simulink model "VFlexP"  (R2024a)
settings: Solver=ode23tb  StartTime=0.0  StopTime=3  FixedStep=1e-5
model workspace (MAT data in the model file):
  DCop_DCBUCK : object (value not decoded)
  Grid_CCVSC_idx = [2; 3; 4; 5; 6; 7; 8; 9; 10; 11; 12]
  Grid_CCVSCs = 1
  Grid_CCVSCs_buses = 1
  Grid_CCVSCs_toM = [0 1 0 0 0 0 0 0 0 0 0 0 ... (781 elements, 71x11)]
  Grid_C_Lines = [0 0]
  Grid_Cbuses = [0.00666666666667 0.00666666666667 0.00666666666667]
  Grid_DC : object (value not decoded)
  Grid_DCop_DCBUCK : object (value not decoded)
  Grid_DCop_DC_PES : object (value not decoded)
  Grid_DFIGs = 1
  Grid_DFIGs_buses = 1
  Grid_DGs : string (value not decoded)
  Grid_From_buses = [1 2]
  Grid_GFls = 1
  Grid_GFls_buses = 1
  Grid_GFr_idx = 1
  Grid_GFrs = 1
  Grid_GFrs_buses = 1
  Grid_GFrs_toM = [1; 0; 0]
  Grid_IG_idx = 2
  Grid_IGs = 1
  Grid_IGs_buses = 1
  Grid_IGs_toM = [0; 1]
  Grid_L_Lines = [0.05 0.05]
  Grid_L_Loads = 0
  Grid_Lines_fromM : object (value not decoded)
  Grid_Lines_toM : object (value not decoded)
  Grid_Load_buses = []
  Grid_Load_busesDC = []
  Grid_MSGs = 1
  Grid_MSGs_buses = 1
  Grid_Nbuses = 3
  Grid_PQ_gen = 3
  Grid_Ploads = []
  Grid_PloadsDC = []
  Grid_Ps_lf = -0.138475313333
  Grid_Qloads = []
  Grid_Qs_lf = 0.00594619333333
  Grid_R_Lines = [0.005 0.005]
  Grid_R_Loads = 0
  Grid_R_Loads_DC = 0
  Grid_Rcf = [150 150 150]
  Grid_SCs = 1
  Grid_SCs_buses = 1
  Grid_SG_idx = 1
  Grid_SGs = 1
  Grid_SGs_buses = 1
  Grid_SGs_toM = [1; 0]
  Grid_To_buses = [2 3]
  Grid_VCVSC_idx = [1; 2; 3; 4; 5; 6; 7; 8; 9; 10; 11; 12]
  Grid_VCVSCs = 1
  Grid_VCVSCs_buses = [1; 2; 3; 6; 8; 9; 12; 58; 59; 60; 63; 65]
  Grid_VCVSCs_toM = [1 0 0 0 0 0 0 0 0 0 0 0 ... (852 elements, 71x12)]
  Grid_VSM_idx = 2
  Grid_VSMs = 1
  Grid_VSMs_buses = 1
  Grid_VSMs_toM = [0; 1]
  Grid_admitt_matrix = [1.9801990198-19.801979198i  -1.9801980198+19.801980198i; -1.9801980198+19.801980198i  1.9801990198-19.801979198i]
  Grid_admitt_matrix_noloads = [1.9801990198-19.801979198i  -1.9801980198+19.801980198i; -1.9801980198+19.801980198i  1.9801990198-19.801979198i]
  Grid_bus = [1; 2; 3]
  Grid_busDC_complexity = 1
  Grid_busDC_complexity_PF = 2
  Grid_bus_complexity = [1 1 1]
  Grid_bus_complexity_PF = [1 1 1]
  Grid_buses_lf = 1
  Grid_conductance_matrix = 0.00666666666667
  Grid_conductance_matrix_noloads = 0.00666666666667
  Grid_fref : object (value not decoded)
  Grid_gen_static_params : mBase (value not decoded)
  Grid_iPs_lf = -7.22150378958
  Grid_iQs_lf = 168.17482109
  Grid_iadmitt_matrix = [250000.001075-249999.987531i  249999.998575-250000.012531i; 249999.998575-250000.012531i  250000.001075-249999.987531i]
  Grid_iadmitt_matrix_noloads = [250000.001075-249999.987531i  249999.998575-250000.012531i; 249999.998575-250000.012531i  250000.001075-249999.987531i]
  Grid_iconductance_matrix = 150
  Grid_iconductance_matrix_noloads = 150
  Grid_init_OK_bool = 1
  Grid_intconv_PF : object (value not decoded)
  Grid_lf_op : op_report (value not decoded)
  Grid_lineDC_complexity = []
  Grid_lineDC_complexity_PF = []
  Grid_line_complexity = [1 1]
  Grid_line_complexity_PF = [3 3]
  Grid_loadDC_complexity = []
  Grid_loadDC_complexity_PF = []
  Grid_load_complexity = []
  Grid_load_complexity_PF = []
  Grid_opDC_CCVSC : object (value not decoded)
  Grid_opDC_VSM : object (value not decoded)
  Grid_opGFr : object (value not decoded)
  Grid_opVCVSC : object (value not decoded)
  Grid_op_CCVSC : object (value not decoded)
  Grid_op_IG : object (value not decoded)
  Grid_op_SG : object (value not decoded)
  Grid_op_VSM : object (value not decoded)
  Grid_shift_lines = [0 0]
  Grid_tap_lines = [1 1]
  Grid_v_buses_mod = [1 1.0001218564 1]
  LinsysParamChangeStruct : Param1 (value not decoded)
  Lline = 0.01
  Rline = 1e-05
  linsys : object (value not decoded)
symbols that are objects in the model workspace (value not decoded): Grid_DCop_DC_PES, Grid_DCop_DCBUCK, Grid_op_CCVSC, Grid_op_IG, Grid_op_SG, Grid_op_VSM, Grid_opDC_CCVSC, Grid_opDC_VSM, Grid_opGFr, Grid_opVCVSC
undefined symbols (not defined in the file or in its folder): block_buses_DC, block_idx, CCVSC_idx, Cf, costs, costs2, DFIGs_nodes, DiscIntNeverNeededParam, entity, Fb, Fi, From_nodes, Grid_op_DFIG, Grid_op_DFIG_PQ, Grid_op_MSG, Grid_op_SC, Grid_op_VCVSC, Kic, Kiv, Kpc, Kpv, last_send, Lc, Lf, m, Matrix_flux_to_i, mD, mp, MSGs_buses, Nbuses_DC, nq, op_VCVSC, Psche, Rc, Rf, rkq1, rkq2, SCs_buses, SCs_nodes, sec_control_structure, set_DG_up, set_extra_satur, set_sending_cost, SGs_buses, SGs_nodes, Tf, To_nodes, VI_L, VI_R, WOF_Tf, xkq1, xkq2
libraries: simulink x447, eeGeneralControl x5
(part 10 of 30)

== system VFlexP/Grid/Dynamic/Generators/SG/Electromagnetic ==
  note: 1) Add Subsystem or Model blocks as valid variant choices.
      | 2) You cannot connect blocks at this level. At simulation, connectivity is automatically
      | determined, based on the active variant and port name matching.
  vsd : Inport
  vsq : Inport  Port=2
  vfd : Inport  Port=3
  ws : Inport  Port=4
  order 2 : Subsystem  VariantControl=order 2
  order 8 : Subsystem  VariantControl=order 8
  order 8 nomatrix : Subsystem  VariantControl=order 1  mask{Lssd_pu=Lssd_pu, Lssq_pu=Lssq_pu, Lmd_pu=Lmd_pu, Lmq_pu=Lmq_pu, Lfd_pu=Lfd_pu, Lkd1_pu=Lkd1_pu, Lkd2_pu=Lkd2_pu, Lkq1_pu=Lkq1_pu, Lkq2_pu=Lkq2_pu, Lkq3_pu=Lkq3_pu}
      mask init:
      | for i=1:length(Lssd_pu)
      |         Lssd = Lssd_pu(i);
      |         Lssq = Lssq_pu(i);
      |         Lmd = Lmd_pu(i);
      |         Lmq = Lmq_pu(i);
      |         Lfd = Lfd_pu(i);
      |         Lkd1 = Lkd1_pu(i);
      |         Lkd2 = Lkd2_pu(i);
      |         Lkq1 = Lkq1_pu(i);
      |         Lkq2 = Lkq2_pu(i);
      |         Lkq3 = Lkq3_pu(i);
      |         Matrix_flux_to_i(:,:,i) = [(0 - (Lfd(i)*Lmd(i)^2 + Lkd2(i)*Lmd(i)^2 - Lmd(i)^3 - Lfd(i)*Lkd1(i)*Lkd2(i))/(2*Lmd(i)^4 - Lkd1(i)*Lmd(i)^3 - 2*Lkd2(i)*Lmd(i)^3 - Lmd(i)^3*Lssd(i) - 2*Lfd(i)*Lmd(i)^3 + Lfd(i)*Lkd1(i)*Lmd(i)^2 + Lfd(i)*Lkd2(i)*Lmd(i)^2 + Lkd1(i)*Lkd2(i)*Lmd(i)^2 + Lfd(i)*Lmd(i)^2*Lssd(i) + Lkd2(i)*Lmd(i)^2*Lssd(i) - Lfd(i)*Lkd1(i)*Lkd2(i)*Lssd(i))),  + 0,  + (0 + (Lkd1(i)*Lmd(i)^2 + Lkd2(i)*Lmd(i)^2 - Lmd(i)^3 - Lkd1(i)*Lkd2(i)*Lmd(i))/(2*Lmd(i)^4 - Lkd1(i)*Lmd(i)^3 - 2*Lkd2(i)*Lmd(i)^3 - Lmd(i)^3*Lssd(i) - 2*Lfd(i)*Lmd(i)^3 + Lfd(i)*Lkd1(i)*Lmd(i)^2 + Lfd(i)*Lkd2(i)*Lmd(i)^2 + Lkd1(i)*Lkd2(i)*Lmd(i)^2 + Lfd(i)*Lmd(i)^2*Lssd(i) + Lkd2(i)*Lmd(i)^2*Lssd(i) - Lfd(i)*Lkd1(i)*Lkd2(i)*Lssd(i))),  + (0 + (Lfd(i)*Lmd(i)^2 + Lkd2(i)*Lmd(i)^2 - Lmd(i)^3 - Lfd(i)*Lkd2(i)*Lmd(i))/(2*Lmd(i)^4 - Lkd1(i)*Lmd(i)^3 - 2*Lkd2(i)*Lmd(i)^3 - Lmd(i)^3*Lssd(i) - 2*Lfd(i)*Lmd(i)^3 + Lfd(i)*Lkd1(i)*Lmd(i)^2 + Lfd(i)*Lkd2(i)*Lmd(i)^2 + Lkd1(i)*Lkd2(i)*Lmd(i)^2 + Lfd(i)*Lmd(i)^2*Lssd(i) + Lkd2(i)*Lmd(i)^2*Lssd(i) - Lfd(i)*Lkd1(i)*Lkd2(i)*Lssd(i))),  + (0 + (Lfd(i)*Lmd(i)^2 - Lfd(i)*Lkd1(i)*Lmd(i))/(2*Lmd(i)^4 - Lkd1(i)*Lmd(i)^3 - 2*Lkd2(i)*Lmd(i)^3 - Lmd(i)^3*Lssd(i) - 2*Lfd(i)*Lmd(i)^3 + Lfd(i)*Lkd1(i)*Lmd(i)^2 + Lfd(i)*Lkd2(i)*Lmd(i)^2 + Lkd1(i)*Lkd2(i)*Lmd(i)^2 + Lfd(i)*Lmd(i)^2*Lssd(i) + Lkd2(i)*Lmd(i)^2*Lssd(i) - Lfd(i)*Lkd1(i)*Lkd2(i)*Lssd(i))),  + 0,  + 0,  + 0, ; 0,  + (0 - (Lkq1(i)*Lmq(i)^2 + Lkq2(i)*Lmq(i)^2 + Lkq3(i)*Lmq(i)^2 - 2*Lmq(i)^3 - Lkq1(i)*Lkq2(i)*Lkq3(i))/(3*Lmq(i)^4 - 2*Lkq2(i)*Lmq(i)^3 - 2*Lkq3(i)*Lmq(i)^3 - 2*Lmq(i)^3*Lssq(i) - 2*Lkq1(i)*Lmq(i)^3 + Lkq1(i)*Lkq2(i)*Lmq(i)^2 + Lkq1(i)*Lkq3(i)*Lmq(i)^2 + Lkq2(i)*Lkq3(i)*Lmq(i)^2 + Lkq1(i)*Lmq(i)^2*Lssq(i) + Lkq2(i)*Lmq(i)^2*Lssq(i) + Lkq3(i)*Lmq(i)^2*Lssq(i) - Lkq1(i)*Lkq2(i)*Lkq3(i)*Lssq(i))),  + 0,  + 0,  + 0,  + (0 - (3*Lmq(i)^3 - 2*Lkq2(i)*Lmq(i)^2 - 2*Lkq3(i)*Lmq(i)^2 - 2*Lkq1(i)*Lmq(i)^2 + Lkq1(i)*Lkq2(i)*Lmq(i) + Lkq1(i)*Lkq3(i)*Lmq(i) + Lkq2(i)*Lkq3(i)*Lmq(i))/(3*Lmq(i)^4 - 2*Lkq2(i)*Lmq(i)^3 - 2*Lkq3(i)*Lmq(i)^3 - 2*Lmq(i)^3*Lssq(i) - 2*Lkq1(i)*Lmq(i)^3 + Lkq1(i)*Lkq2(i)*Lmq(i)^2 + Lkq1(i)*Lkq3(i)*Lmq(i)^2 + Lkq2(i)*Lkq3(i)*Lmq(i)^2 + Lkq1(i)*Lmq(i)^2*Lssq(i) + Lkq2(i)*Lmq(i)^2*Lssq(i) + Lkq3(i)*Lmq(i)^2*Lssq(i) - Lkq1(i)*Lkq2(i)*Lkq3(i)*Lssq(i))),  + 0,  + 0, ; (0 - (Lkd2(i)*Lmd(i)^2 - Lkd1(i)*Lkd2(i)*Lmd(i))/(2*Lmd(i)^4 - Lkd1(i)*Lmd(i)^3 - 2*Lkd2(i)*Lmd(i)^3 - Lmd(i)^3*Lssd(i) - 2*Lfd(i)*Lmd(i)^3 + Lfd(i)*Lkd1(i)*Lmd(i)^2 + Lfd(i)*Lkd2(i)*Lmd(i)^2 + Lkd1(i)*Lkd2(i)*Lmd(i)^2 + Lfd(i)*Lmd(i)^2*Lssd(i) + Lkd2(i)*Lmd(i)^2*Lssd(i) - Lfd(i)*Lkd1(i)*Lkd2(i)*Lssd(i))),  + 0,  + (0 + (Lkd1(i)*Lmd(i)^2 + Lkd2(i)*Lmd(i)^2 + Lmd(i)^2*Lssd(i) - 2*Lmd(i)^3 - Lkd1(i)*Lkd2(i)*Lssd(i))/(2*Lmd(i)^4 - Lkd1(i)*Lmd(i)^3 - 2*Lkd2(i)*Lmd(i)^3 - Lmd(i)^3*Lssd(i) - 2*Lfd(i)*Lmd(i)^3 + Lfd(i)*Lkd1(i)*Lmd(i)^2 + Lfd(i)*Lkd2(i)*Lmd(i)^2 + Lkd1(i)*Lkd2(i)*Lmd(i)^2 + Lfd(i)*Lmd(i)^2*Lssd(i) + Lkd2(i)*Lmd(i)^2*Lssd(i) - Lfd(i)*Lkd1(i)*Lkd2(i)*Lssd(i))),  + (0 - (Lkd2(i)*Lmd(i)^2 - Lkd2(i)*Lssd(i)*Lmd(i))/(2*Lmd(i)^4 - Lkd1(i)*Lmd(i)^3 - 2*Lkd2(i)*Lmd(i)^3 - Lmd(i)^3*Lssd(i) - 2*Lfd(i)*Lmd(i)^3 + Lfd(i)*Lkd1(i)*Lmd(i)^2 + Lfd(i)*Lkd2(i)*Lmd(i)^2 + Lkd1(i)*Lkd2(i)*Lmd(i)^2 + Lfd(i)*Lmd(i)^2*Lssd(i) + Lkd2(i)*Lmd(i)^2*Lssd(i) - Lfd(i)*Lkd1(i)*Lkd2(i)*Lssd(i))),  + (0 - (Lkd1(i)*Lmd(i)^2 + Lmd(i)^2*Lssd(i) - 2*Lmd(i)^3)/(2*Lmd(i)^4 - Lkd1(i)*Lmd(i)^3 - 2*Lkd2(i)*Lmd(i)^3 - Lmd(i)^3*Lssd(i) - 2*Lfd(i)*Lmd(i)^3 + Lfd(i)*Lkd1(i)*Lmd(i)^2 + Lfd(i)*Lkd2(i)*Lmd(i)^2 + Lkd1(i)*Lkd2(i)*Lmd(i)^2 + Lfd(i)*Lmd(i)^2*Lssd(i) + Lkd2(i)*Lmd(i)^2*Lssd(i) - Lfd(i)*Lkd1(i)*Lkd2(i)*Lssd(i))),  + 0,  + 0,  + 0, ; (0 - (Lfd(i)*Lmd(i)^2 + Lkd2(i)*Lmd(i)^2 - Lmd(i)^3 - Lfd(i)*Lkd2(i)*Lmd(i))/(2*Lmd(i)^4 - Lkd1(i)*Lmd(i)^3 - 2*Lkd2(i)*Lmd(i)^3 - Lmd(i)^3*Lssd(i) - 2*Lfd(i)*Lmd(i)^3 + Lfd(i)*Lkd1(i)*Lmd(i)^2 + Lfd(i)*Lkd2(i)*Lmd(i)^2 + Lkd1(i)*Lkd2(i)*Lmd(i)^2 + Lfd(i)*Lmd(i)^2*Lssd(i) + Lkd2(i)*Lmd(i)^2*Lssd(i) - Lfd(i)*Lkd1(i)*Lkd2(i)*Lssd(i))),  + 0,  + (0 - (Lkd2(i)*Lmd(i)^2 + Lmd(i)^2*Lssd(i) - Lmd(i)^3 - Lkd2(i)*Lmd(i)*Lssd(i))/(2*Lmd(i)^4 - Lkd1(i)*Lmd(i)^3 - 2*Lkd2(i)*Lmd(i)^3 - Lmd(i)^3*Lssd(i) - 2*Lfd(i)*Lmd(i)^3 + Lfd(i)*Lkd1(i)*Lmd(i)^2 + Lfd(i)*Lkd2(i)*Lmd(i)^2 + Lkd1(i)*Lkd2(i)*Lmd(i)^2 + Lfd(i)*Lmd(i)^2*Lssd(i) + Lkd2(i)*Lmd(i)^2*Lssd(i) - Lfd(i)*Lkd1(i)*Lkd2(i)*Lssd(i))),  + (0 + (Lfd(i)*Lmd(i)^2 + Lkd2(i)*Lmd(i)^2 - Lmd(i)^3 - Lfd(i)*Lkd2(i)*Lssd(i))/(2*Lmd(i)^4 - Lkd1(i)*Lmd(i)^3 - 2*Lkd2(i)*Lmd(i)^3 - Lmd(i)^3*Lssd(i) - 2*Lfd(i)*Lmd(i)^3 + Lfd(i)*Lkd1(i)*Lmd(i)^2 + Lfd(i)*Lkd2(i)*Lmd(i)^2 + Lkd1(i)*Lkd2(i)*Lmd(i)^2 + Lfd(i)*Lmd(i)^2*Lssd(i) + Lkd2(i)*Lmd(i)^2*Lssd(i) - Lfd(i)*Lkd1(i)*Lkd2(i)*Lssd(i))),  + (0 - (Lfd(i)*Lmd(i)^2 - Lfd(i)*Lssd(i)*Lmd(i))/(2*Lmd(i)^4 - Lkd1(i)*Lmd(i)^3 - 2*Lkd2(i)*Lmd(i)^3 - Lmd(i)^3*Lssd(i) - 2*Lfd(i)*Lmd(i)^3 + Lfd(i)*Lkd1(i)*Lmd(i)^2 + Lfd(i)*Lkd2(i)*Lmd(i)^2 + Lkd1(i)*Lkd2(i)*Lmd(i)^2 + Lfd(i)*Lmd(i)^2*Lssd(i) + Lkd2(i)*Lmd(i)^2*Lssd(i) - Lfd(i)*Lkd1(i)*Lkd2(i)*Lssd(i))),  + 0,  + 0,  + 0, ; (0 - (Lfd(i)*Lmd(i)^2 + Lkd1(i)*Lmd(i)^2 - Lmd(i)^3 - Lfd(i)*Lkd1(i)*Lmd(i))/(2*Lmd(i)^4 - Lkd1(i)*Lmd(i)^3 - 2*Lkd2(i)*Lmd(i)^3 - Lmd(i)^3*Lssd(i) - 2*Lfd(i)*Lmd(i)^3 + Lfd(i)*Lkd1(i)*Lmd(i)^2 + Lfd(i)*Lkd2(i)*Lmd(i)^2 + Lkd1(i)*Lkd2(i)*Lmd(i)^2 + Lfd(i)*Lmd(i)^2*Lssd(i) + Lkd2(i)*Lmd(i)^2*Lssd(i) - Lfd(i)*Lkd1(i)*Lkd2(i)*Lssd(i))),  + 0,  + (0 - (Lkd1(i)*Lmd(i)^2 + Lmd(i)^2*Lssd(i) - Lmd(i)^3 - Lkd1(i)*Lmd(i)*Lssd(i))/(2*Lmd(i)^4 - Lkd1(i)*Lmd(i)^3 - 2*Lkd2(i)*Lmd(i)^3 - Lmd(i)^3*Lssd(i) - 2*Lfd(i)*Lmd(i)^3 + Lfd(i)*Lkd1(i)*Lmd(i)^2 + Lfd(i)*Lkd2(i)*Lmd(i)^2 + Lkd1(i)*Lkd2(i)*Lmd(i)^2 + Lfd(i)*Lmd(i)^2*Lssd(i) + Lkd2(i)*Lmd(i)^2*Lssd(i) - Lfd(i)*Lkd1(i)*Lkd2(i)*Lssd(i))),  + (0 - (Lfd(i)*Lmd(i)^2 + Lmd(i)^2*Lssd(i) - Lmd(i)^3 - Lfd(i)*Lmd(i)*Lssd(i))/(2*Lmd(i)^4 - Lkd1(i)*Lmd(i)^3 - 2*Lkd2(i)*Lmd(i)^3 - Lmd(i)^3*Lssd(i) - 2*Lfd(i)*Lmd(i)^3 + Lfd(i)*Lkd1(i)*Lmd(i)^2 + Lfd(i)*Lkd2(i)*Lmd(i)^2 + Lkd1(i)*Lkd2(i)*Lmd(i)^2 + Lfd(i)*Lmd(i)^2*Lssd(i) + Lkd2(i)*Lmd(i)^2*Lssd(i) - Lfd(i)*Lkd1(i)*Lkd2(i)*Lssd(i))),  + (0 + (Lfd(i)*Lmd(i)^2 + Lkd1(i)*Lmd(i)^2 + Lmd(i)^2*Lssd(i) - 2*Lmd(i)^3 - Lfd(i)*Lkd1(i)*Lssd(i))/(2*Lmd(i)^4 - Lkd1(i)*Lmd(i)^3 - 2*Lkd2(i)*Lmd(i)^3 - Lmd(i)^3*Lssd(i) - 2*Lfd(i)*Lmd(i)^3 + Lfd(i)*Lkd1(i)*Lmd(i)^2 + Lfd(i)*Lkd2(i)*Lmd(i)^2 + Lkd1(i)*Lkd2(i)*Lmd(i)^2 + Lfd(i)*Lmd(i)^2*Lssd(i) + Lkd2(i)*Lmd(i)^2*Lssd(i) - Lfd(i)*Lkd1(i)*Lkd2(i)*Lssd(i))),  + 0,  + 0,  + 0, ; 0,  + (0 - (Lkq2(i)*Lmq(i)^2 + Lkq3(i)*Lmq(i)^2 - Lmq(i)^3 - Lkq2(i)*Lkq3(i)*Lmq(i))/(3*Lmq(i)^4 - 2*Lkq2(i)*Lmq(i)^3 - 2*Lkq3(i)*Lmq(i)^3 - 2*Lmq(i)^3*Lssq(i) - 2*Lkq1(i)*Lmq(i)^3 + Lkq1(i)*Lkq2(i)*Lmq(i)^2 + Lkq1(i)*Lkq3(i)*Lmq(i)^2 + Lkq2(i)*Lkq3(i)*Lmq(i)^2 + Lkq1(i)*Lmq(i)^2*Lssq(i) + Lkq2(i)*Lmq(i)^2*Lssq(i) + Lkq3(i)*Lmq(i)^2*Lssq(i) - Lkq1(i)*Lkq2(i)*Lkq3(i)*Lssq(i))),  + 0,  + 0,  + 0,  + (0 - (Lmq(i)^2*Lssq(i) + Lkq2(i)*Lkq3(i)*Lssq(i) - Lkq2(i)*Lmq(i)*Lssq(i) - Lkq3(i)*Lmq(i)*Lssq(i))/(3*Lmq(i)^4 - 2*Lkq2(i)*Lmq(i)^3 - 2*Lkq3(i)*Lmq(i)^3 - 2*Lmq(i)^3*Lssq(i) - 2*Lkq1(i)*Lmq(i)^3 + Lkq1(i)*Lkq2(i)*Lmq(i)^2 + Lkq1(i)*Lkq3(i)*Lmq(i)^2 + Lkq2(i)*Lkq3(i)*Lmq(i)^2 + Lkq1(i)*Lmq(i)^2*Lssq(i) + Lkq2(i)*Lmq(i)^2*Lssq(i) + Lkq3(i)*Lmq(i)^2*Lssq(i) - Lkq1(i)*Lkq2(i)*Lkq3(i)*Lssq(i))),  + 0,  + 0, ; 0,  + (0 + (Lmq(i)*(Lkq1(i) - Lmq(i))*(Lkq3(i) - Lmq(i)))/(3*Lmq(i)^4 - 2*Lkq2(i)*Lmq(i)^3 - 2*Lkq3(i)*Lmq(i)^3 - 2*Lmq(i)^3*Lssq(i) - 2*Lkq1(i)*Lmq(i)^3 + Lkq1(i)*Lkq2(i)*Lmq(i)^2 + Lkq1(i)*Lkq3(i)*Lmq(i)^2 + Lkq2(i)*Lkq3(i)*Lmq(i)^2 + Lkq1(i)*Lmq(i)^2*Lssq(i) + Lkq2(i)*Lmq(i)^2*Lssq(i) + Lkq3(i)*Lmq(i)^2*Lssq(i) - Lkq1(i)*Lkq2(i)*Lkq3(i)*Lssq(i))),  + 0,  + 0,  + 0,  + (0 - (Lssq(i)*(Lkq1(i) - Lmq(i))*(Lkq3(i) - Lmq(i)))/(3*Lmq(i)^4 - 2*Lkq2(i)*Lmq(i)^3 - 2*Lkq3(i)*Lmq(i)^3 - 2*Lmq(i)^3*Lssq(i) - 2*Lkq1(i)*Lmq(i)^3 + Lkq1(i)*Lkq2(i)*Lmq(i)^2 + Lkq1(i)*Lkq3(i)*Lmq(i)^2 + Lkq2(i)*Lkq3(i)*Lmq(i)^2 + Lkq1(i)*Lmq(i)^2*Lssq(i) + Lkq2(i)*Lmq(i)^2*Lssq(i) + Lkq3(i)*Lmq(i)^2*Lssq(i) - Lkq1(i)*Lkq2(i)*Lkq3(i)*Lssq(i))),  + 0,  + 0, ; 0,  + (0 + (Lmq(i)*(Lkq1(i) - Lmq(i))*(Lkq2(i) - Lmq(i)))/(3*Lmq(i)^4 - 2*Lkq2(i)*Lmq(i)^3 - 2*Lkq3(i)*Lmq(i)^3 - 2*Lmq(i)^3*Lssq(i) - 2*Lkq1(i)*Lmq(i)^3 + Lkq1(i)*Lkq2(i)*Lmq(i)^2 + Lkq1(i)*Lkq3(i)*Lmq(i)^2 + Lkq2(i)*Lkq3(i)*Lmq(i)^2 + Lkq1(i)*Lmq(i)^2*Lssq(i) + Lkq2(i)*Lmq(i)^2*Lssq(i) + Lkq3(i)*Lmq(i)^2*Lssq(i) - Lkq1(i)*Lkq2(i)*Lkq3(i)*Lssq(i))),  + 0,  + 0,  + 0,  + (0 - (Lssq(i)*(Lkq1(i) - Lmq(i))*(Lkq2(i) - Lmq(i)))/(3*Lmq(i)^4 - 2*Lkq2(i)*Lmq(i)^3 - 2*Lkq3(i)*Lmq(i)^3 - 2*Lmq(i)^3*Lssq(i) - 2*Lkq1(i)*Lmq(i)^3 + Lkq1(i)*Lkq2(i)*Lmq(i)^2 + Lkq1(i)*Lkq3(i)*Lmq(i)^2 + Lkq2(i)*Lkq3(i)*Lmq(i)^2 + Lkq1(i)*Lmq(i)^2*Lssq(i) + Lkq2(i)*Lmq(i)^2*Lssq(i) + Lkq3(i)*Lmq(i)^2*Lssq(i) - Lkq1(i)*Lkq2(i)*Lkq3(i)*Lssq(i))),  + 0,  + 0, ];
      |     end
  isd : Outport
  isq : Outport  Port=2
  psi : Outport  Port=3

== system VFlexP/Grid/Dynamic/Generators/SG/For Each Subsystem ==
  In1 : Inport  Partition=on  PartitionDimension=1  PartitionWidth=1  PartitionOffset=0
  For Each : ForEach  DisableCoverage=on
  State-Space : StateSpace  A=[]  B=[]  C=[]  D=block_toM  InitialCondition=0  ParameterTunability=Optimized
  Transpose : Math  Operator=transpose
  Transpose1 : Math  Operator=transpose
  Out1 : Outport  ConcatenationDimension=1
  wires:
  Transpose1/1 -> Out1/1
  In1/1 -> Transpose/1
  Transpose/1 -> State-Space/1
  State-Space/1 -> Transpose1/1

== system VFlexP/Grid/Dynamic/Generators/SG/LPF2 ==
  in : Inport
  Gain : Gain  Gain=1./T_s
  Sum4 : Sum  Inputs=|+-
  x_a : Integrator  InitialCondition=Grid_op_SG.op.States(4).x'
  out : Outport
  wires:
  Gain/1 -> x_a/1
  Sum4/1 -> Gain/1
  in/1 -> Sum4/1
  x_a/1 -> out/1, Sum4/2

== system VFlexP/Grid/Dynamic/Generators/SG/LPF4 ==
  in : Inport
  Gain : Gain  Gain=1./T_s
  Sum4 : Sum  Inputs=|+-
  x_a : Integrator  InitialCondition=Grid_op_SG.op.States(10).x'
  out : Outport
  wires:
  x_a/1 -> Sum4/2, out/1
  in/1 -> Sum4/1
  Sum4/1 -> Gain/1
  Gain/1 -> x_a/1

== system VFlexP/Grid/Dynamic/Generators/SG/LPF5 ==
  in : Inport
  Gain : Gain  Gain=1./T_s
  Sum4 : Sum  Inputs=|+-
  x_a : Integrator  InitialCondition=Grid_op_SG.op.States(11).x'
  out : Outport
  wires:
  Gain/1 -> x_a/1
  Sum4/1 -> Gain/1
  in/1 -> Sum4/1
  x_a/1 -> out/1, Sum4/2

== system VFlexP/Grid/Dynamic/Generators/SG/PIv_d1 ==
  In1 : Inport
  Gain : Gain  Gain=10
  Gain1 : Gain  Gain=200
  I : Integrator  InitialCondition=Grid_op_SG.op.States(7).x'
  Sum10 : Sum  Inputs=|++
  vfd : Outport
  wires:
  In1/1 -> Gain1/1, Gain/1
  Sum10/1 -> vfd/1
  Gain/1 -> Sum10/1
  I/1 -> Sum10/2
  Gain1/1 -> I/1

== system VFlexP/Grid/Dynamic/Generators/SG/Reference frame transform1 ==
  in_d : Inport
  theta : Inport  Port=2
  in_q : Inport  Port=3
  Complex to Real-Imag : ComplexToRealImag
  Cos : Trigonometry  SCDEnableBlockLinearizationSpecification=on  Operator=cos
  Product : Product
  Real-Imag to Complex : RealImagToComplex
  Real-Imag to Complex1 : RealImagToComplex
  Sin : Trigonometry  SCDEnableBlockLinearizationSpecification=on
  out_d : Outport
  out_q : Outport  Port=2
  wires:
  in_d/1 -> Real-Imag to Complex/1
  in_q/1 -> Real-Imag to Complex/2
  Complex to Real-Imag/1 -> out_d/1
  Sin/1 -> Real-Imag to Complex1/2
  Cos/1 -> Real-Imag to Complex1/1
  theta/1 -> Cos/1, Sin/1
  Product/1 -> Complex to Real-Imag/1
  Real-Imag to Complex/1 -> Product/2
  Real-Imag to Complex1/1 -> Product/1
  Complex to Real-Imag/2 -> out_q/1

== system VFlexP/Grid/Dynamic/Generators/SG/Reference frame transform3 ==
  in_d : Inport
  theta : Inport  Port=2
  in_q : Inport  Port=3
  Complex to Real-Imag : ComplexToRealImag
  Cos : Trigonometry  SCDEnableBlockLinearizationSpecification=on  Operator=cos
  Product : Product
  Real-Imag to Complex : RealImagToComplex
  Real-Imag to Complex1 : RealImagToComplex
  Sin : Trigonometry  SCDEnableBlockLinearizationSpecification=on
  out_d : Outport
  out_q : Outport  Port=2
  wires:
  Complex to Real-Imag/2 -> out_q/1
  Real-Imag to Complex1/1 -> Product/1
  Real-Imag to Complex/1 -> Product/2
  Product/1 -> Complex to Real-Imag/1
  theta/1 -> Sin/1, Cos/1
  Cos/1 -> Real-Imag to Complex1/1
  Sin/1 -> Real-Imag to Complex1/2
  Complex to Real-Imag/1 -> out_d/1
  in_q/1 -> Real-Imag to Complex/2
  in_d/1 -> Real-Imag to Complex/1

== system VFlexP/Grid/Dynamic/Generators/SG/Rotor axis ==
  te : Inport
  tm : Inport  Port=2
  Gain : Gain  Gain=1/2./H
  Gain1 : Gain  Gain=D
  Sum1 : Sum  Inputs=+|-|-  InputSameDT=on  SaturateOnIntegerOverflow=on  OutDataTypeStr=Inherit: Same as first input
  \omega_r : Integrator  InitialCondition=Grid_op_SG.op.States(7).x'  UpperSaturationLimit=2*pi  LowerSaturationLimit=0
  wr : Outport  VectorParamsAs1DForOutWhenUnconnected=off
  wires:
  tm/1 -> Sum1/1
  \omega_r/1 -> wr/1, Gain1/1
  te/1 -> Sum1/2
  Sum1/1 -> Gain/1
  Gain/1 -> \omega_r/1
  Gain1/1 -> Sum1/3

== system VFlexP/Grid/Dynamic/Generators/SG/Subsystem2 ==
  In1 : Inport
  Gain : Gain  Gain=1./T_1
  Gain2 : Gain  Gain=T_2./T_1
  Sum : Sum  Inputs=|+-
  Sum1 : Sum  Inputs=++|
  x_f : Integrator  InitialCondition=Grid_op_SG.op.States(17).x'
  Out1 : Outport
  wires:
  x_f/1 -> Sum1/2, Sum/2
  Gain/1 -> x_f/1
  Sum/1 -> Gain/1, Gain2/1
  Gain2/1 -> Sum1/1
  Sum1/1 -> Out1/1
  In1/1 -> Sum/1

== system VFlexP/Grid/Dynamic/Generators/SG/Subsystem4 ==
  In1 : Inport
  Gain : Gain  Gain=1./T_1
  Gain2 : Gain  Gain=T_2./T_1
  Sum : Sum  Inputs=|+-
  Sum1 : Sum  Inputs=++|
  x_f : Integrator  InitialCondition=Grid_op_SG.op.States(18).x'
  Out1 : Outport
  wires:
  x_f/1 -> Sum1/2, Sum/2
  Gain/1 -> x_f/1
  Sum/1 -> Gain/1, Gain2/1
  Gain2/1 -> Sum1/1
  Sum1/1 -> Out1/1
  In1/1 -> Sum/1

== system VFlexP/Grid/Dynamic/Generators/SG/Torque ==
  psi : Inport
  isd : Inport  Port=2
  isq : Inport  Port=3
  Product1 : Product
  Product2 : Product
  Selector : Selector  NumberOfDimensions=2  InputPortWidth=9  IndexOptions=Index vector (dialog),Select all  Indices=[1],1  OutputSizes=1,1
  Selector1 : Selector  NumberOfDimensions=2  InputPortWidth=9  IndexOptions=Index vector (dialog),Select all  Indices=[2],1  OutputSizes=1,1
  Sum : Sum  Inputs=+||-
  te : Outport  VectorParamsAs1DForOutWhenUnconnected=off
  wires:
  Product1/1 -> Sum/1
  Sum/1 -> te/1
  Selector/1 -> Product1/1  "psistatordq"
  psi/1 -> Selector1/1, Selector/1
  Product2/1 -> Sum/2
  isq/1 -> Product1/2
  isd/1 -> Product2/1
  Selector1/1 -> Product2/2  "psistatordq"

== system VFlexP/Grid/Dynamic/Generators/SG/connect ==
  id : Inport
  iq : Inport  Port=2
  connect : Inport  Port=3
  Switch : Switch  Criteria=u2 > Threshold  ZeroCross=off  SaturateOnIntegerOverflow=off  InputSameDT=off
  Switch1 : Switch  Criteria=u2 > Threshold  ZeroCross=off  SaturateOnIntegerOverflow=off  InputSameDT=off
  Zero1 : Constant  Value=0  VectorParams1D=off  OutDataTypeStr=Inherit: Inherit via back propagation
  Zero2 : Constant  Value=0  VectorParams1D=off  OutDataTypeStr=Inherit: Inherit via back propagation
  id_real : Outport
  iq_real : Outport  Port=2
  connected : Outport  Port=3  OutDataTypeStr=boolean
  wires:
  Switch/1 -> id_real/1
  Zero1/1 -> Switch/3
  id/1 -> Switch/1
  connect/1 -> connected/1, Switch1/2, Switch/2
  Switch1/1 -> iq_real/1
  iq/1 -> Switch1/1
  Zero2/1 -> Switch1/3

== system VFlexP/Grid/Dynamic/Generators/SG/trim_output ==
  id : Inport
  iq : Inport  Port=2
  vd : Inport  Port=3
  vq : Inport  Port=4
  Out1 : Outport
  Out2 : Outport  Port=2
  Out3 : Outport  Port=3
  Out4 : Outport  Port=4
  wires:
  id/1 -> Out1/1
  vq/1 -> Out4/1
  vd/1 -> Out3/1
  iq/1 -> Out2/1

== system VFlexP/Grid/Dynamic/Generators/VSM/For Each Subsystem ==
  In1 : Inport  Partition=on  PartitionDimension=1  PartitionWidth=1  PartitionOffset=0
  For Each : ForEach  DisableCoverage=on
  State-Space : StateSpace  A=[]  B=[]  C=[]  D=block_toM  InitialCondition=0  ParameterTunability=Optimized
  Transpose : Math  Operator=transpose
  Transpose1 : Math  Operator=transpose
  Out1 : Outport  ConcatenationDimension=1
  wires:
  In1/1 -> Transpose/1
  Transpose1/1 -> Out1/1
  Transpose/1 -> State-Space/1
  State-Space/1 -> Transpose1/1

== system VFlexP/Grid/Dynamic/Generators/VSM/LPF1 ==
  In1 : Inport
  Gain : Gain  Gain=1e2
  I : Integrator  InitialCondition=Grid_op_VSM.op.States(2).x'
  Sum4 : Sum  Inputs=|+-
  Out1 : Outport
  wires:
  I/1 -> Sum4/2, Out1/1
  In1/1 -> Sum4/1
  Sum4/1 -> Gain/1
  Gain/1 -> I/1

== system VFlexP/Grid/Dynamic/Generators/VSM/LPF4 ==
  In1 : Inport
  Gain : Gain  Gain=1e2
  I : Integrator  InitialCondition=Grid_op_VSM.op.States(3).x'
  Sum4 : Sum  Inputs=|+-
  Out1 : Outport
  wires:
  Gain/1 -> I/1
  Sum4/1 -> Gain/1
  In1/1 -> Sum4/1
  I/1 -> Out1/1, Sum4/2

== system VFlexP/Grid/Dynamic/Generators/VSM/LPF5 ==
  In1 : Inport
  Gain : Gain  Gain=1e2
  I : Integrator  InitialCondition=Grid_op_VSM.op.States(4).x'
  Sum4 : Sum  Inputs=|+-
  Out1 : Outport
  wires:
  I/1 -> Sum4/2, Out1/1
  In1/1 -> Sum4/1
  Sum4/1 -> Gain/1
  Gain/1 -> I/1

== system VFlexP/Grid/Dynamic/Generators/VSM/PC ==
  ioq : Inport
  iodi : Inport  Port=2
  Eref : Inport  Port=3
  vodi : Inport  Port=4
  voq : Inport  Port=5
  omegasp : Inport  Port=6
  Psp : Inport  Port=7
  Divide : Product  Inputs=*/
  Gain : Gain  Gain=1./Rv
  Gain1 : Gain  Gain=Dv
  Gain2 : Gain  Gain=1./(2*Hv)
  Integrator : Integrator  InitialCondition=Grid_op_VSM.op.States(3).x'
  Integrator1 : Integrator  InitialCondition=Grid_op_VSM.op.States(4).x'
  LPF_P : Subsystem
  LPF_Q : Subsystem
  P : InitialCondition  Commented=through
  Product{,1..3} (4 alike) : Product
  Q : InitialCondition  Commented=through
  Sum : Sum  Inputs=|++
  Sum1 : Sum  Inputs=|-+
  Sum2 : Sum  Inputs=|++
  Sum3 : Sum  Inputs=|-+
  Sum4 : Sum  Inputs=+|+|+
  Sum5 : Sum  Inputs=+-|
  Sum6 : Sum  Inputs=|+-
  Sum7 : Sum  Inputs=|+-
  Turbine model : Subsystem
  WOF_d : Subsystem  Commented=through
  Zero : Constant  Value=0  OutDataTypeStr=Inherit: Inherit via back propagation
  nq1 : Gain  Gain=nq
  omega : Outport
  Out2 : Outport  Port=2
  P_f : Outport  Port=3
  Q_f : Outport  Port=4
  wires:
  ioq/1 -> Product1/2, Product2/2  "ioq"
  iodi/1 -> Product/2, Product3/2  "iod"
  voq/1 -> Product3/1, Product1/1  "voq"
  Sum1/1 -> Q/1
  Sum/1 -> P/1
  LPF_Q/1(Q_f) -> nq1/1, Q_f/1
  LPF_P/1(P_f) -> P_f/1, Sum6/2
  Sum3/1 -> Out2/1  "vodref"
  Eref/1 -> Sum3/2  "Eref"
  nq1/1 -> Sum3/1  "nqQ"
  Product3/1 -> Sum1/2
  Product2/1 -> Sum1/1
  Product1/1 -> Sum/2
  Product/1 -> Sum/1
  vodi/1 -> Product/1, Product2/1  "vod"
  P/1 -> LPF_P/1(P)
  Q/1 -> LPF_Q/1(Q)
  omegasp/1 -> Sum5/1
  Sum5/1 -> Gain/1
  Sum4/1 -> Turbine model/1(In1)
  Sum7/1 -> Gain2/1
  Gain2/1 -> Integrator/1
  Integrator/1 -> WOF_d/1(In1), Sum2/1
  Zero/1 -> Sum2/2
  WOF_d/1(Out1) -> Gain1/1
  Gain1/1 -> Sum7/2
  Psp/1 -> Sum4/2
  Turbine model/1(Out1) -> Sum6/1
  Sum6/1 -> Divide/1
  Divide/1 -> Sum7/1
  Sum2/1 -> omega/1, Sum5/2, Divide/2
  Integrator1/1 -> Sum4/3
  Gain/1 -> Sum4/1

== system VFlexP/Grid/Dynamic/Generators/VSM/PI ==
  In1 : Inport
  Gain : Gain  Gain=0.1
  Gain1 : Gain  Gain=0.2
  I : Integrator  InitialCondition=Grid_op_VSM.op.States(7).x'
  Sum10 : Sum  Inputs=|++
  Out1 : Outport
  wires:
  In1/1 -> Gain1/1, Gain/1
  Sum10/1 -> Out1/1
  Gain/1 -> Sum10/1
  I/1 -> Sum10/2
  Gain1/1 -> I/1

== system VFlexP/Grid/Dynamic/Generators/VSM/PI1 ==
  In1 : Inport
  Gain : Gain  Gain=0.1/100/pi
  Gain1 : Gain  Gain=0.2/100/pi
  I : Integrator  InitialCondition=Grid_op_VSM.op.States(8).x'
  Sum10 : Sum  Inputs=|++
  Out1 : Outport
  wires:
  Gain1/1 -> I/1
  I/1 -> Sum10/2
  Gain/1 -> Sum10/1
  Sum10/1 -> Out1/1
  In1/1 -> Gain/1, Gain1/1

== system VFlexP/Grid/Dynamic/Generators/VSM/RL out ==
  note: 1) Add Subsystem or Model blocks as valid variant choices.
      | 2) You cannot connect blocks at this level. At simulation, connectivity is automatically
      | determined, based on the active variant and port name matching.
  v_in_d : Inport
  v_out_d : Inport  Port=2
  v_in_q : Inport  Port=3
  v_out_q : Inport  Port=4
  dynamic : Subsystem  VariantControl=dynamic
  static : Subsystem  VariantControl=static
  static_omega : Subsystem  VariantControl=static_omega
  id : Outport
  iq : Outport  Port=2
  v_outd : Outport  Port=3
  v_outq : Outport  Port=4

== system VFlexP/Grid/Dynamic/Generators/VSM/Reference frame transform1 ==
  in_d : Inport
  theta : Inport  Port=2
  in_q : Inport  Port=3
  Complex to Real-Imag : ComplexToRealImag
  Cos : Trigonometry  SCDEnableBlockLinearizationSpecification=on  Operator=cos
  Product : Product
  Real-Imag to Complex : RealImagToComplex
  Real-Imag to Complex1 : RealImagToComplex
  Sin : Trigonometry  SCDEnableBlockLinearizationSpecification=on
  out_d : Outport
  out_q : Outport  Port=2
  wires:
  in_d/1 -> Real-Imag to Complex/1
  in_q/1 -> Real-Imag to Complex/2
  Complex to Real-Imag/1 -> out_d/1
  Sin/1 -> Real-Imag to Complex1/2
  Cos/1 -> Real-Imag to Complex1/1
  theta/1 -> Cos/1, Sin/1
  Product/1 -> Complex to Real-Imag/1
  Real-Imag to Complex/1 -> Product/2
  Real-Imag to Complex1/1 -> Product/1
  Complex to Real-Imag/2 -> out_q/1

== system VFlexP/Grid/Dynamic/Generators/VSM/Reference frame transform2 ==
  in_d : Inport
  theta : Inport  Port=2
  in_q : Inport  Port=3
  Complex to Real-Imag : ComplexToRealImag
  Cos : Trigonometry  SCDEnableBlockLinearizationSpecification=on  Operator=cos
  Product : Product
  Real-Imag to Complex : RealImagToComplex
  Real-Imag to Complex1 : RealImagToComplex
  Sin : Trigonometry  SCDEnableBlockLinearizationSpecification=on
  out_d : Outport
  out_q : Outport  Port=2
  wires:
  Complex to Real-Imag/2 -> out_q/1
  Real-Imag to Complex1/1 -> Product/1
  Real-Imag to Complex/1 -> Product/2
  Product/1 -> Complex to Real-Imag/1
  theta/1 -> Sin/1, Cos/1
  Cos/1 -> Real-Imag to Complex1/1
  Sin/1 -> Real-Imag to Complex1/2
  Complex to Real-Imag/1 -> out_d/1
  in_q/1 -> Real-Imag to Complex/2
  in_d/1 -> Real-Imag to Complex/1

== system VFlexP/Grid/Dynamic/Generators/VSM/Reference frame transform3 ==
  in_d : Inport
  theta : Inport  Port=2
  in_q : Inport  Port=3
  Complex to Real-Imag : ComplexToRealImag
  Cos : Trigonometry  SCDEnableBlockLinearizationSpecification=on  Operator=cos
  Product : Product
  Real-Imag to Complex : RealImagToComplex
  Real-Imag to Complex1 : RealImagToComplex
  Sin : Trigonometry  SCDEnableBlockLinearizationSpecification=on
  out_d : Outport
  out_q : Outport  Port=2
  wires:
  in_d/1 -> Real-Imag to Complex/1
  in_q/1 -> Real-Imag to Complex/2
  Complex to Real-Imag/1 -> out_d/1
  Sin/1 -> Real-Imag to Complex1/2
  Cos/1 -> Real-Imag to Complex1/1
  theta/1 -> Sin/1, Cos/1
  Product/1 -> Complex to Real-Imag/1
  Real-Imag to Complex/1 -> Product/2
  Real-Imag to Complex1/1 -> Product/1
  Complex to Real-Imag/2 -> out_q/1

== system VFlexP/Grid/Dynamic/Generators/VSM/VCC ==
  note: 1) Add Subsystem or Model blocks as valid variant choices.
      | 2) You cannot connect blocks at this level. At simulation, connectivity is automatically
      | determined, based on the active variant and port name matching.
  vodref : Inport
  voqref : Inport  Port=2
  iod : Inport  Port=3
  ioq : Inport  Port=4
  omega : Inport  Port=5
  dynamic : Subsystem  VariantControl=dynamic
  dynamic_VC : Subsystem  VariantControl=dynamic_VC
  dynamic_limiting : Subsystem  VariantControl=dynamic_limiting
  static : Subsystem  VariantControl=static
  vidref : Outport
  viqref : Outport  Port=2

== system VFlexP/Grid/Dynamic/Generators/VSM/VI ==
  id : Inport
  iq : Inport  Port=2
  omega : Inport  Port=3
  Gain : Gain  Gain=L
  Gain1 : Gain  Gain=R
  Gain2 : Gain  Gain=L
  Gain3 : Gain  Gain=R
  Product : Product
  Product1 : Product
  Sum : Sum  Inputs=-+|
  Sum1 : Sum  Inputs=|--
  WOF_d : Subsystem
  WOF_q : Subsystem
  vd : Outport
  vq : Outport  Port=2
  wires:
  Gain/1 -> Product/1
  omega/1 -> Product/2, Product1/1
  iq/1 -> WOF_q/1(In1)
  Product/1 -> Sum/2
  id/1 -> WOF_d/1(In1)
  Gain2/1 -> Product1/2
  Product1/1 -> Sum1/1
  Gain1/1 -> Sum/1
  Gain3/1 -> Sum1/2
  Sum/1 -> vd/1
  Sum1/1 -> vq/1
  WOF_d/1(Out1) -> Gain2/1, Gain1/1
  WOF_q/1(Out1) -> Gain3/1, Gain/1

== system VFlexP/Grid/Dynamic/Generators/VSM/connect ==
  id : Inport
  iq : Inport  Port=2
  connect : Inport  Port=3
  Switch : Switch  Criteria=u2 > Threshold  ZeroCross=off  SaturateOnIntegerOverflow=off  InputSameDT=off
  Switch1 : Switch  Criteria=u2 > Threshold  ZeroCross=off  SaturateOnIntegerOverflow=off  InputSameDT=off
  Zero1 : Constant  Value=0  VectorParams1D=off  OutDataTypeStr=Inherit: Inherit via back propagation
  Zero2 : Constant  Value=0  VectorParams1D=off  OutDataTypeStr=Inherit: Inherit via back propagation
  id_real : Outport
  iq_real : Outport  Port=2
  connected : Outport  Port=3  OutDataTypeStr=boolean
  wires:
  Zero2/1 -> Switch1/3
  iq/1 -> Switch1/1
  Switch1/1 -> iq_real/1
  connect/1 -> Switch/2, Switch1/2, connected/1
  id/1 -> Switch/1
  Zero1/1 -> Switch/3
  Switch/1 -> id_real/1

== system VFlexP/Grid/Dynamic/Generators/VSM/trim_output ==
  id : Inport
  iq : Inport  Port=2
  vd : Inport  Port=3
  vq : Inport  Port=4
  Out1 : Outport
  Out2 : Outport  Port=2
  Out3 : Outport  Port=3
  Out4 : Outport  Port=4
  wires:
  iq/1 -> Out2/1
  vd/1 -> Out3/1
  vq/1 -> Out4/1
  id/1 -> Out1/1

== system VFlexP/Grid/Dynamic/Grid/Dynamic/Buses ==
  i_in : Inport
  i_out : Inport  Port=2
  Sum : Sum  Inputs=|++++
  dynamic : Subsystem  VariantControl=dynamic
  only R : Subsystem  Commented=on  VariantControl=only R
  static : Subsystem  Commented=on  VariantControl=static
  static omega : Subsystem  Commented=on  VariantControl=static omega
  v : Outport
  wires:
  static omega/1(v) -> Sum/3
  i_out/1 -> only R/2(i_out), static omega/2(i_out), static/2(i_out), dynamic/2(i_out)
  dynamic/1(v) -> Sum/1
  i_in/1 -> only R/1(i_in), static omega/1(i_in), static/1(i_in), dynamic/1(i_in)
  only R/1(v) -> Sum/4
  static/1(v) -> Sum/2
  Sum/1 -> v/1

== system VFlexP/Grid/Dynamic/Grid/Dynamic/Lines ==
  v_in : Inport
  v_out : Inport  Port=2
  connected : Inport  Port=3
  Constant1 : Constant  Value=zeros(1, length(R_Lines))  VectorParams1D=off
  Matrix Concatenate : Concatenate  NumInputs=3  Mode=Multidimensional array
  Selector : Selector  NumberOfDimensions=2  InputPortWidth=3  IndexOptions=Index vector (dialog),Select all  Indices=1,1  OutputSizes=1,1
  Selector1 : Selector  NumberOfDimensions=2  InputPortWidth=3  IndexOptions=Index vector (dialog),Select all  Indices=2,1  OutputSizes=1,1
  Sum : Sum  Inputs=|+++
  dynamic : Subsystem  VariantControl=dynamic
  static : Subsystem  Commented=on  VariantControl=static
  static omega : Subsystem  Commented=on  VariantControl=static_omega
  tap transformer : Subsystem
  i : Outport
  wires:
  connected/1 -> static omega/3(connected), static/3(connected), dynamic/3(connected)
  v_out/1 -> static omega/2(v_out), static/2(v_out_d), dynamic/2(v_out)
  Matrix Concatenate/1 -> dynamic/1(v_in_d), static omega/1(v_in_d), static/1(v_in)
  dynamic/1(i) -> Sum/1
  static/1(i) -> Sum/2
  static omega/1(i) -> Sum/3
  Sum/1 -> i/1
  v_in/1 -> Selector1/1, Selector/1
  Selector/1 -> tap transformer/1(in_d)
  Selector1/1 -> tap transformer/2(in_q)
  Constant1/1 -> Matrix Concatenate/3
  tap transformer/1(out_d) -> Matrix Concatenate/1
  tap transformer/2(out_q) -> Matrix Concatenate/2

== system VFlexP/Grid/Dynamic/Grid/Dynamic/Lines to buses ==
  i : Inport
  Complex to Real-Imag : ComplexToRealImag
  Constant1 : Constant  Value=zeros(1, length(R_Lines))  VectorParams1D=off
  Gain : Gain  Gain=1./tap_lines.*(cos(shift_lines)-1i*sin(shift_lines))
  Lines_toM : Subsystem  TreatAsAtomicUnit=on
  Matrix Concatenate : Concatenate  NumInputs=3  Mode=Multidimensional array
  Real-Imag to Complex : RealImagToComplex
  Selector : Selector  NumberOfDimensions=2  InputPortWidth=3  IndexOptions=Index vector (dialog),Select all  Indices=1,1  OutputSizes=1,1
  Selector1 : Selector  NumberOfDimensions=2  InputPortWidth=3  IndexOptions=Index vector (dialog),Select all  Indices=2,1  OutputSizes=1,1
  i_in_buses : Outport
  i_out_buses : Outport  Port=2
  wires:
  Lines_toM/2(i_to_lines) -> i_out_buses/1
  i/1 -> Lines_toM/1(i_to), Selector1/1, Selector/1
  Lines_toM/1(i_from_lines) -> i_in_buses/1
  Matrix Concatenate/1 -> Lines_toM/2(i_from)
  Real-Imag to Complex/1 -> Gain/1
  Selector1/1 -> Real-Imag to Complex/2
  Selector/1 -> Real-Imag to Complex/1
  Complex to Real-Imag/1 -> Matrix Concatenate/1
  Complex to Real-Imag/2 -> Matrix Concatenate/2
  Gain/1 -> Complex to Real-Imag/1
  Constant1/1 -> Matrix Concatenate/3

== system VFlexP/Grid/Dynamic/Grid/Dynamic/Loads ==
  v_in : Inport
  connected : Inport  Port=2
  iP : Inport  Port=3
  PQ : Subsystem  Commented=on  VariantControl=PQ
  Sum : Sum  Inputs=|++++++++
  dynamic PQ : Subsystem  Commented=on  VariantControl=dynamic_PQ
  parallel RL dynamic : Subsystem  Commented=on  VariantControl=dynamic
  parallel RL static : Subsystem  Commented=on  VariantControl=dynamic
  parallel RL static omega : Subsystem  Commented=on  VariantControl=dynamic
  series RL dynamic : Subsystem  Commented=on  VariantControl=dynamic
  series RL static : Subsystem  Commented=on  VariantControl=static
  series RL static omega : Subsystem  Commented=on  VariantControl=static_omega
  i : Outport
  wires:
  v_in/1 -> series RL dynamic/1(v_in), parallel RL dynamic/1(v_in), parallel RL static omega/1(v_in), parallel RL static/1(v_in), dynamic PQ/1(v_in), PQ/1(v_in), series RL static omega/1(v_in), series RL static/2(v_in)
  series RL dynamic/1(i) -> Sum/1
  connected/1 -> series RL dynamic/2(connected), parallel RL dynamic/2(connected), parallel RL static omega/2(connected), parallel RL static/2(connected), dynamic PQ/2(connected), PQ/2(connected), series RL static omega/2(connected), series RL static/1(connected)
  iP/1 -> PQ/3(iP), dynamic PQ/3(iP)
  series RL static/1(i) -> Sum/2
  PQ/1(i) -> Sum/4
  dynamic PQ/1(i) -> Sum/5
  series RL static omega/1(i) -> Sum/3
  Sum/1 -> i/1
  parallel RL dynamic/1(i) -> Sum/6
  parallel RL static/1(i) -> Sum/7
  parallel RL static omega/1(i) -> Sum/8

== system VFlexP/Grid/Dynamic/Grid/Dynamic/Loads to buses ==
  i_loads : Inport
  LoadsM : Subsystem  TreatAsAtomicUnit=on
  i_out_buses : Outport
  wires:
  i_loads/1 -> LoadsM/1(i)
  LoadsM/1(Out1) -> i_out_buses/1

== system VFlexP/Grid/Dynamic/Grid/Dynamic/connect ==
  note: in which load?
      | By default, the max(P)
  Assignment : Assignment  DiagnosticForDimensions=Warning  IndexOptions=Index vector (dialog)  Indices=1  OutputSizes=1
  One3 : Constant  Value=ones(1, length(L_Loads))  VectorParams1D=off  OutDataTypeStr=Inherit: Inherit via back propagation
  Step : Step  Before=1  SampleTime=0
  Out1 : Outport
  wires:
  Assignment/1 -> Out1/1
  One3/1 -> Assignment/1
  Step/1 -> Assignment/2

== system VFlexP/Grid/Dynamic/Grid/Dynamic/iCbuses ==
  In1 : Inport
  Constant : Constant  Value=Cbuses  VectorParams1D=off
  Constant1 : Constant  Value=C_Lines  VectorParams1D=off
  Gain : Gain  Gain=1/2
  Saturation : Saturate  UpperLimit=inf  LowerLimit=1e-3
  Subsystem : Subsystem
  Sum3 : Sum  Inputs=|-+
  Switch : Switch  Criteria=u2 > Threshold  SaturateOnIntegerOverflow=off  InputSameDT=off
  Zero : Constant  Value=zeros(1, length(From_buses))  VectorParams1D=off  OutDataTypeStr=Inherit: Inherit via back propagation
  Out1 : Outport
  wires:
  Switch/1 -> Gain/1
  Sum3/1 -> Saturation/1
  Zero/1 -> Switch/1
  Saturation/1 -> Out1/1
  Constant/1 -> Sum3/2
  Gain/1 -> Subsystem/1(In1)
  Constant1/1 -> Switch/3
  In1/1 -> Switch/2
  Subsystem/1(Out1) -> Sum3/1

== system VFlexP/Grid/Dynamic/Grid/Dynamic/iP ==
  note: in which load?
      | By default, the max(P)
  Assignment : Assignment  DiagnosticForDimensions=Warning  IndexOptions=Index vector (dialog)  Indices=find(Ploads == max(Ploads), 1)  OutputSizes=1
  Gain : Gain  Gain=0
  One3 : Constant  Value=zeros(1, length(L_Loads))  VectorParams1D=off  OutDataTypeStr=Inherit: Inherit via back propagation
  iP in % : Step  After=0.1  SampleTime=0  VectorParams1D=off  ZeroCross=off
  Out1 : Outport
  wires:
  One3/1 -> Assignment/1
  iP in %/1 -> Gain/1
  Assignment/1 -> Out1/1
  Gain/1 -> Assignment/2

== system VFlexP/Grid/Dynamic/Grid_DC/dynamic/BusesDC ==
  Input : Inport
  Input1 : Inport  Port=2
  Sum : Sum
  dynamic : Subsystem
  static : Subsystem  Commented=on
  v : Outport
  wires:
  Input/1 -> static/1(i_in), dynamic/1(i_in)
  Input1/1 -> static/2(i_out), dynamic/2(i_out)
  dynamic/1(v) -> Sum/1
  static/1(v) -> Sum/2
  Sum/1 -> v/1

== system VFlexP/Grid/Dynamic/Grid_DC/dynamic/DC_Lines_toM1 ==
  i : Inport
  State-Space : StateSpace  A=[]  B=[]  C=[]  D=DC.Lines_toM  InitialCondition=0  ParameterTunability=Optimized
  State-Space1 : StateSpace  A=[]  B=[]  C=[]  D=DC.Lines_fromM  InitialCondition=0  ParameterTunability=Optimized
  Transpose{,1..3} (4 alike) : Math  Operator=transpose
  i_from_lines : Outport
  i_to_lines : Outport  Port=2
  wires:
  Transpose2/1 -> ?
  i/1 -> Transpose2/1, Transpose/1
  Transpose3/1 -> i_to_lines/1
  Transpose/1 -> ?
  State-Space1/1 -> Transpose3/1
  State-Space/1 -> Transpose1/1
  Transpose1/1 -> i_from_lines/1

== system VFlexP/Grid/Dynamic/Grid_DC/dynamic/DClines ==
  V_dc_In : Inport
  V_dc_out : Inport  Port=2
  Dynamic : Subsystem  Commented=on
  Static : Subsystem  Commented=on
  Sum4 : Sum
  i : Outport
  wires:
  V_dc_In/1 -> Static/1(V_dc_In), Dynamic/1(V_dc_In)
  V_dc_out/1 -> Dynamic/2(V_dc_Out), Static/2(V_dc_Out)
  Dynamic/1(i) -> Sum4/1
  Static/1(i) -> Sum4/2
  Sum4/1 -> i/1

== system VFlexP/Grid/Dynamic/Grid_DC/dynamic/Loads ==
  v_in : Inport
  connected : Inport  Port=2
  ConstI : Subsystem  Commented=on
  ConstP : Subsystem  Commented=on
  ConstR : Subsystem  Commented=on
  DynamicP : Subsystem  Commented=on
  Sum4 : Sum  Inputs=++++
  i : Outport
  wires:
  ConstR/1(i) -> Sum4/2
  ConstP/1(i) -> Sum4/1
  connected/1 -> DynamicP/2(connected), ConstI/1(connected), ConstR/2(connected), ConstP/2(connected)
  v_in/1 -> DynamicP/1(v_in), ConstR/1(v_in), ConstP/1(v_in)
  Sum4/1 -> i/1
  ConstI/1(i) -> Sum4/3
  DynamicP/1(i) -> Sum4/4

== system VFlexP/Grid/Dynamic/Grid_DC/dynamic/Loads to buses ==
  i_loads : Inport
  LoadsM : Subsystem  TreatAsAtomicUnit=on
  i_out_buses : Outport
  wires:
  i_loads/1 -> LoadsM/1(i)
  LoadsM/1(i_out_buses) -> i_out_buses/1

== system VFlexP/Grid/Dynamic/Grid_DC/static/LPF_d1 ==
  In1 : Inport
  Gain : Gain  Gain=1000
  I : Integrator  InitialCondition=DC.v
  Sum4 : Sum  Inputs=|+-
  v_buses_dc : Outport
  wires:
  Sum4/1 -> Gain/1
  In1/1 -> Sum4/1
  I/1 -> v_buses_dc/1, Sum4/2
  Gain/1 -> I/1
